simulink model "bnbPid_Simulink"  (R2026a)
settings: Solver=VariableStepAuto  StopTime=10
undefined symbols (not defined in the file): K_BB
libraries: slpidlib x1
settings Model: Creator=Paul Oh  LastModifiedBy=user

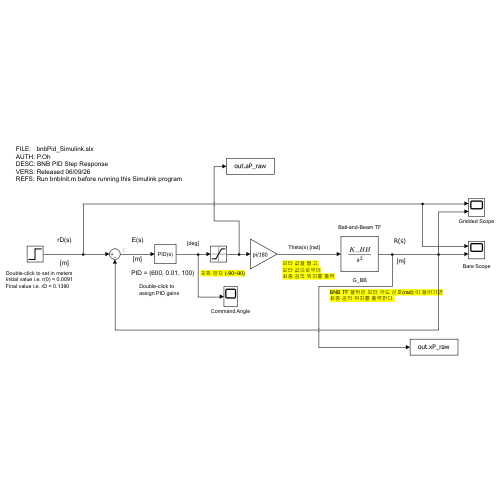
[thumbnail: Simulink's stored preview of the top-level diagram]
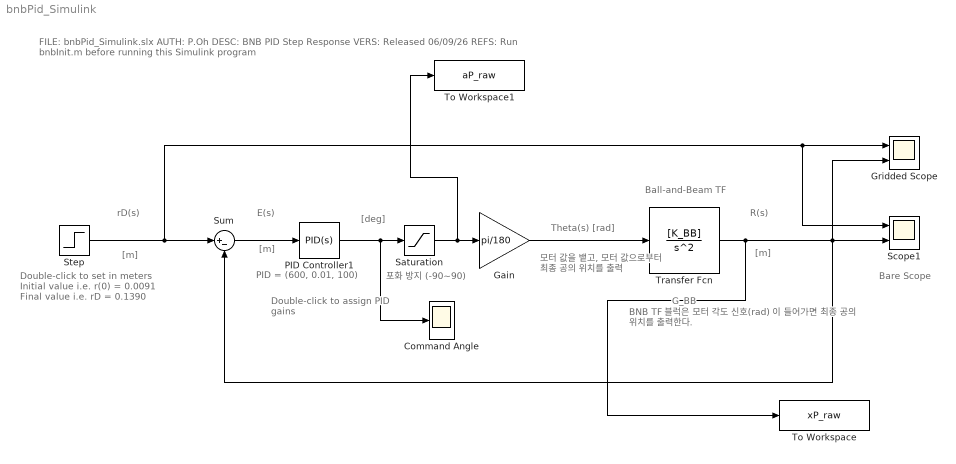
== system bnbPid_Simulink ==
  note: 모터 값을 뱉고,
      | 모터 값으로부터
      | 최종 공의 위치를 출력
  note: 포화 방지 (-90~90)
  note: Double-click to assign PID gains
  note: Bare Scope
  note: Theta(s) [rad]
  note: [deg]
  note: Double-click to set in meters
      | Initial value i.e. r(0) = 0.0091
      | Final value i.e. rD = 0.1390
  note: Ball-and-Beam TF
  note: [m]
  note: rD(s)
  note: [m]
  note: E(s)
  note: R(s)
  note: [m]
  note: PID = (600, 0.01, 100)
  note: FILE: bnbPid_Simulink.slx
      | AUTH: P.Oh
      | DESC: BNB PID Step Response
      | VERS: Released 06/09/26
      | REFS: Run bnbInit.m before running this Simulink program
  note: G_BB
  note: BNB TF 블럭은 모터 각도 신호(rad) 이 들어가면
      | 최종 공의 위치를 출력한다.
  Command Angle : Scope
      settings: ActiveDisplayYMinimum=-241.60130291599211  ActiveDisplayYMaximum=1663.9557003239993
  Gain : Gain  Gain=pi/180
  Gridded Scope : Scope  NumInputPorts=2
      settings: SampleTime=0.02  ActiveDisplayYMinimum=-0.027282275035775492  ActiveDisplayYMaximum=0.24554047532197948
  PID Controller1 : slpidlib/PID Controller  Controller=PID  Form=Parallel  TimeDomain=Continuous-time  UseExternalTs=off  SampleTime=-1  IntegratorMethod=Forward Euler  FilterMethod=Forward Euler  ControllerParametersSource=internal  P=600  I=0.01  UseKiTs=off  D=100  UseExternalDerivativeSource=off  N=100  UseFilter=on  TunerSelectOption=Transfer Function Based (PID Tuner App)  InitialConditionSource=internal  InitialConditionForIntegrator=0  InitialConditionForFilter=0  DifferentiatorICPrevScaledInput=0  ExternalReset=none  TrackingMode=off  Kt=1  LimitOutput=off  SatLimitsSource=internal  UpperSaturationLimit=inf  LowerSaturationLimit=-inf  LinearizeAsGain=on  AntiWindupMode=none  Kb=1  LimitIntegrator=off  UpperIntegratorSaturationLimit=inf  LowerIntegratorSaturationLimit=-inf  POutMin=[]  POutMax=[]  IOutMin=[]  IOutMax=[]  DOutMin=[]  DOutMax=[]  NOutMin=[]  NOutMax=[]  SumOutMin=[]  SumOutMax=[]  SaturationOutMin=[]  SaturationOutMax=[]  PParamMin=[]  PParamMax=[]  IParamMin=[]  IParamMax=[]  DParamMin=[]  DParamMax=[]  NParamMin=[]  NParamMax=[]  KbParamMin=[]  KbParamMax=[]  KtParamMin=[]  KtParamMax=[]  KbOutMin=[]  KbOutMax=[]  KtOutMin=[]  KtOutMax=[]  IntegratorOutMin=[]  IntegratorOutMax=[]  FilterOutMin=[]  FilterOutMax=[]  SumI1OutMin=[]  SumI1OutMax=[]  SumI2OutMin=[]  SumI2OutMax=[]  SumI3OutMin=[]  SumI3OutMax=[]  SumI4OutMin=[]  SumI4OutMax=[]  SumDOutMin=[]  SumDOutMax=[]  DifferentiatorOutMin=[]  DifferentiatorOutMax=[]  FilterDiffOutCoefMin=[]  FilterDiffOutCoefMax=[]  ReciprocalOutMin=[]  ReciprocalOutMax=[]  SumDenOutMin=[]  SumDenOutMax=[]  SumNumOutMin=[]  SumNumOutMax=[]  DivideOutMin=[]  DivideOutMax=[]  UdiffTsProdOutMin=[]  UdiffTsProdOutMax=[]  NTsProdOutMin=[]  NTsProdOutMax=[]  UintegralTsProdOutMin=[]  UintegralTsProdOutMax=[]  UngainTsProdOutMin=[]  UngainTsProdOutMax=[]  ClampingZeroOutDataTypeStr=Inherit: Inherit via back propagation  ClampingZeroOutMin=[]  ClampingZeroOutMax=[]  FilterDenConstantOutDataTypeStr=Inherit: Inherit via back propagation  FilterDenConstantOutMin=[]  FilterDenConstantOutMax=[]  PCopyOutDataTypeStr=Inherit: Inherit via back propagation  PCopyOutMin=[]  PCopyOutMax=[]  NCopyOutDataTypeStr=Inherit: Inherit via back propagation  NCopyOutMin=[]  NCopyOutMax=[]  IntegratorContinuousStateAttributes=''  IntegratorStateMustResolveToSignalObject=off  IntegratorRTWStateStorageClass=Auto  FilterContinuousStateAttributes=''  FilterStateMustResolveToSignalObject=off  FilterRTWStateStorageClass=Auto  ParallelPVariant=InternalParameters  IdealPVariant=Disabled  IVariant=InternalParameters  DVariant=InternalParameters  IntegratorVariant=Continuous  SatVariant=Disabled  AWVariant=Passthrough  PCopyVariant=Disabled  TRVariant=Disabled  FdbkBlocksVariant=Forward  IdealPFdbkVariant=Disabled  SatFdbkVariant=Disabled  DerivativeFilterVariant=ContFilter  NVariant=InternalParameters  NCopyVariant=Disabled  FilterICVariant=InternalICsFilter  IntegratorICVariant=InternalICs  ExternalResetVariant=Disabled  TRSumVariant=Passthrough  SumFdbkVariant=Disabled  SumVariant=Sum_PID  TsampFilterVariant=InternalTs  TsampNgainVariant=Passthrough  TsampIntegralVariant=Disabled_SignalSpec  ExternalSaturationOutDataTypeStr=Inherit: Same as second input  DerivativeSourceVariant=ErrorSignal  PreIntVariant=InternalPreInt
  Saturation : Saturate  UpperLimit=30  LowerLimit=-30
  Scope1 : Scope  NumInputPorts=2
      settings: ActiveDisplayYMinimum=-0.027282275035775492  ActiveDisplayYMaximum=0.24554047532197948
  Step : Step  Time=0.0  FinalValue=0.1  SampleTime=0.0020
  Sum : Sum  Inputs=|+-
  To Workspace : ToWorkspace  VariableName=xP_raw  SaveFormat=Timeseries  SampleTime=-1
  To Workspace1 : ToWorkspace  VariableName=aP_raw  SaveFormat=Timeseries  SampleTime=-1
  Transfer Fcn : TransferFcn  Numerator=[K_BB]  Denominator=[1 0 0]
  wires:
  Sum/1 -> PID Controller1/1
  Step/1 -> Scope1/1, Gridded Scope/1, Sum/1
  PID Controller1/1 -> Saturation/1, Command Angle/1
  Saturation/1 -> To Workspace1/1, Gain/1
  Transfer Fcn/1 -> To Workspace/1, Gridded Scope/2, Sum/2, Scope1/2
  Gain/1 -> Transfer Fcn/1
